simulink model "hps"  (R2021b)
settings: Solver=FixedStepAuto  StartTime=0.0  StopTime=20  FixedStep=0.00909  MaxStep=0.01  RelTol=1e-4  EnableMultiTasking=on
libraries: simulink_extras x5, slpidlib x3, vrlib x3, aerolibutil x2, shared6dof x1, sharedutil x1, sharedtransform x1
settings Model: Creator=rizo  LastModifiedBy=rizo
settings DataIOCC: LimitDataPoints=on  SaveOutput=off  SaveTime=off
settings OptimizationCC: ExpressionDepthLimit=2147483647  LifeSpan=1
settings DebuggingCC: UnderspecifiedInitializationDetection=Classic  MergeDetectMultiDrivingBlocksExec=none  AllowSymbolicDim=off  StateNameClashWarn=warning  SFUnexpectedBacktrackingDiag=warning  SFNoUnconditionalDefaultTransitionDiag=warning  SFExecutionAtInitializationDiag=none  SFMachineParentedDataDiag=warning  ArithmeticOperatorsInVariantConditions=warning
settings SFSimCC: SimUseLocalCustomCode=off  CustomCodeUndefinedFunction=UseInterfaceOnly
settings RTWCC: RTWUseLocalCustomCode=off
settings CodeAppCC: StateflowObjectComments=on
settings GRTTargetCC: TargetLangStandard=C89/C90 (ANSI)  CombineOutputUpdateFcns=off  GRTInterface=on

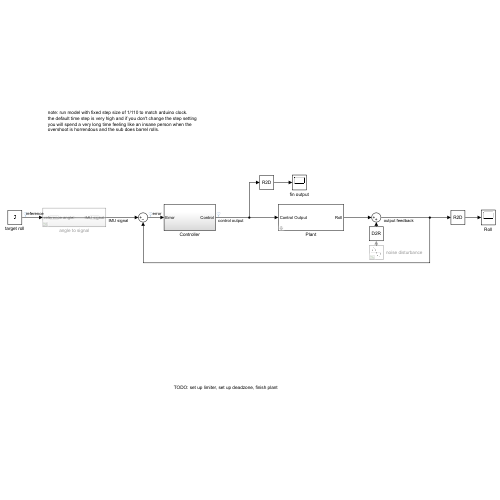
[thumbnail: Simulink's stored preview of the top-level diagram]
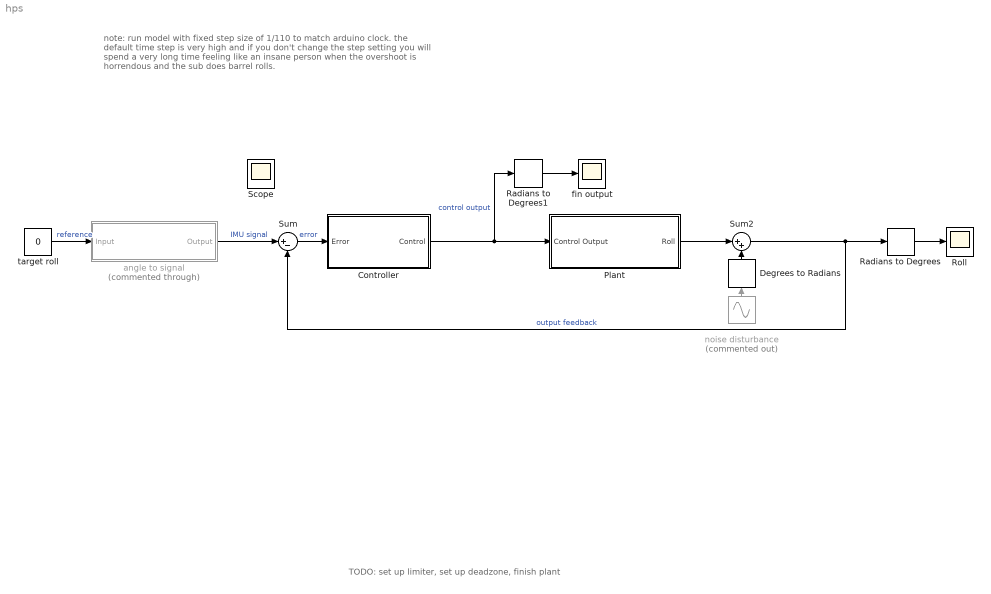
== system hps ==
  note: note: run model with fixed step size of 1/110 to match arduino clock.
      | the default time step is very high and if you don't change the step setting
      | you will spend a very long time feeling like an insane person when the
      | overshoot is horrendous and the sub does barrel rolls.
  note: TODO: set up limiter, set up deadzone, finish plant
  Controller : Subsystem
  Degrees to Radians : simulink_extras/Transformations/Degrees to Radians
  Plant : Subsystem  mask{initial_velocity=1.5, initial_roll=pi/180 * 15, mass=121, Ig=[11.5 -16.5 -21.6; -16.5 165 -3.54; -21.6 -3.54 162], pedaling=10, acc=.25}
      mask prompts: initial_velocity "Initial Velocity"; initial_roll "Initial Roll Angle"; mass "Submarine Mass"; Ig "Inertia matrix"; pedaling "Pedaling Disturbance (N)"; acc "Accerleration (m/s^2)"
  Radians to Degrees : simulink_extras/Transformations/Radians to Degrees
  Radians to Degrees1 : simulink_extras/Transformations/Radians to Degrees
  Roll : Scope
  Sum : Sum  Inputs=|+-
  Sum2 : Sum  Inputs=|++
  angle to signal : Subsystem  Commented=through
  fin output : Scope
  noise disturbance : Sin  Commented=on  Amplitude=0  SampleTime=0
  target roll : Constant  Value=0
  Scope : Scope
  wires:
  target roll/1 -> angle to signal/1(Input)  "reference"
  Sum/1 -> Controller/1(Error)  "error"
  Controller/1(Control) -> Plant/1(Control Output), Radians to Degrees1/1  "control output"
  Sum2/1 -> Sum/2, Radians to Degrees/1  "output feedback"
  angle to signal/1(Output) -> Sum/1  "IMU signal"
  Plant/1(Roll) -> Sum2/1
  Radians to Degrees1/1 -> fin output/1
  Radians to Degrees/1 -> Roll/1
  Degrees to Radians/1 -> Sum2/2
  noise disturbance/1 -> Degrees to Radians/1

== system hps/Controller ==
  Error : Inport
  Controller V0.1 : Subsystem  Commented=on
  Controller V0.2 : Subsystem
  Steering Gear : TransferFcn  Denominator=[1 1]
  Control : Outport
  wires:
  Error/1 -> Controller V0.1/1(Error), Controller V0.2/1(Error)
  Controller V0.2/1(Control) -> Steering Gear/1
  Steering Gear/1 -> Control/1

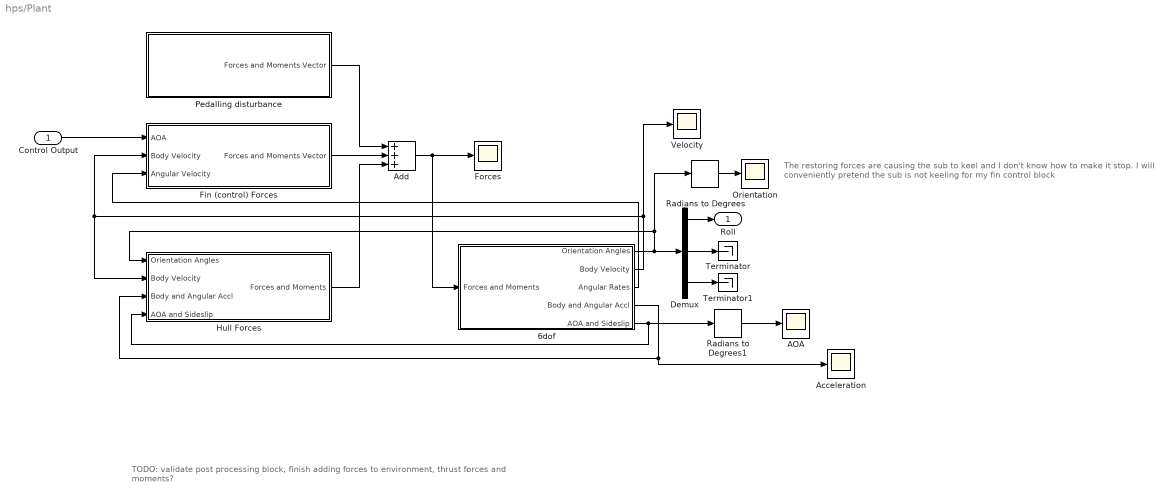
== system hps/Plant ==
  note: The restoring forces are causing the sub to keel and I don't know how to make it stop. I will conveniently pretend the sub is not keeling for my fin control block
  note: TODO: validate post processing block, finish adding forces to environment, thrust forces and moments?
  Control Output : Inport
  6dof : Subsystem
  AOA : Scope
  Acceleration : Scope
  Add : Sum  Inputs=+++
  Demux : Demux  Outputs=3
  Fin (control) Forces : Subsystem  mask{r=.405, finbeam=1.37, semi_major=48.64, semi_minor=12.34, cd=1.28, cl=.108, A=.0942, ro=997}
      mask prompts: r "Fin radius from center"; finbeam "Fin beam"; semi_major "Semi-major axis"; semi_minor "Semi-minor axis"; cd "Coefficient of Drag"; cl "Coefficient of Lift"; A "Planform Area of Wing (m^2)"; ro "Density of Water (kg/m^3)"
  Forces : Scope
  Hull Forces : Subsystem
  Orientation : Scope
  Pedalling disturbance : Subsystem  mask{f=pedaling, a=acc}
      mask prompts: f "Pedal Force (N)"; a "Acceleration (m/s^2)"
  Radians to Degrees : simulink_extras/Transformations/Radians to Degrees
  Radians to Degrees1 : simulink_extras/Transformations/Radians to Degrees
  Terminator : Terminator
  Terminator1 : Terminator
  Velocity : Scope
  Roll : Outport
  wires:
  Control Output/1 -> Fin (control) Forces/1(AOA)
  6dof/1(Orientation Angles) -> Demux/1, Radians to Degrees/1, Hull Forces/1(Orientation Angles)
  Hull Forces/1(Forces and Moments) -> Add/3
  Demux/1 -> Roll/1
  Demux/2 -> Terminator/1
  Demux/3 -> Terminator1/1
  6dof/2(Body Velocity) -> Velocity/1, Hull Forces/2(Body Velocity), Fin (control) Forces/2(Body Velocity)
  Fin (control) Forces/1(Forces and Moments Vector) -> Add/2
  Add/1 -> Forces/1, 6dof/1(Forces and Moments)
  6dof/3(Angular Rates) -> Fin (control) Forces/3(Angular Velocity)
  Pedalling disturbance/1(Forces and Moments Vector) -> Add/1
  6dof/5(AOA and Sideslip) -> Hull Forces/4(AOA and Sideslip), Radians to Degrees1/1
  6dof/4(Body and Angular Accl) -> Acceleration/1, Hull Forces/3(Body and Angular Accl)
  Radians to Degrees/1 -> Orientation/1
  Radians to Degrees1/1 -> AOA/1

== system hps/angle to signal ==
  Input : Inport
  Gain : Gain
  Output : Outport
  wires:
  Gain/1 -> Output/1  "IMU signal"
  Input/1 -> Gain/1  "reference angle"

== system hps/Controller/Controller V0.1 ==
  Error : Inport
  Dead Zone1 : DeadZone  LowerValue=-pi/180 * 2  UpperValue=pi/180 * 2  SaturateOnIntegerOverflow=on
  Dead Zone2 : DeadZone  LowerValue=-pi/180 * 2  UpperValue=pi/180 * 2  SaturateOnIntegerOverflow=on
  PI Controller : slpidlib/PID Controller  Controller=PID  Form=Parallel  TimeDomain=Continuous-time  UseExternalTs=off  SampleTime=-1  IntegratorMethod=Forward Euler  FilterMethod=Forward Euler  ControllerParametersSource=internal  P=4  I=1  D=0  UseFilter=on  N=100  TunerSelectOption=Transfer Function Based (PID Tuner App)  InitialConditionSource=internal  InitialConditionForIntegrator=0  InitialConditionForFilter=0  DifferentiatorICPrevScaledInput=0  ExternalReset=none  TrackingMode=off  Kt=1  LimitOutput=off  SatLimitsSource=internal  UpperSaturationLimit=inf  LowerSaturationLimit=-inf  LinearizeAsGain=on  AntiWindupMode=none  Kb=1  POutMin=[]  POutMax=[]  IOutMin=[]  IOutMax=[]  DOutMin=[]  DOutMax=[]  NOutMin=[]  NOutMax=[]  SumOutMin=[]  SumOutMax=[]  SaturationOutMin=[]  SaturationOutMax=[]  PParamMin=[]  PParamMax=[]  IParamMin=[]  IParamMax=[]  DParamMin=[]  DParamMax=[]  NParamMin=[]  NParamMax=[]  KbParamMin=[]  KbParamMax=[]  KtParamMin=[]  KtParamMax=[]  KbOutMin=[]  KbOutMax=[]  KtOutMin=[]  KtOutMax=[]  IntegratorOutMin=[]  IntegratorOutMax=[]  FilterOutMin=[]  FilterOutMax=[]  SumI1OutMin=[]  SumI1OutMax=[]  SumI2OutMin=[]  SumI2OutMax=[]  SumI3OutMin=[]  SumI3OutMax=[]  SumI4OutMin=[]  SumI4OutMax=[]  SumDOutMin=[]  SumDOutMax=[]  DifferentiatorOutMin=[]  DifferentiatorOutMax=[]  FilterDiffOutCoefMin=[]  FilterDiffOutCoefMax=[]  ReciprocalOutMin=[]  ReciprocalOutMax=[]  SumDenOutMin=[]  SumDenOutMax=[]  SumNumOutMin=[]  SumNumOutMax=[]  DivideOutMin=[]  DivideOutMax=[]  UdiffTsProdOutMin=[]  UdiffTsProdOutMax=[]  NTsProdOutMin=[]  NTsProdOutMax=[]  UintegralTsProdOutMin=[]  UintegralTsProdOutMax=[]  UngainTsProdOutMin=[]  UngainTsProdOutMax=[]  IntegratorContinuousStateAttributes=''  IntegratorStateMustResolveToSignalObject=off  IntegratorRTWStateStorageClass=Auto  FilterContinuousStateAttributes=''  FilterStateMustResolveToSignalObject=off  FilterRTWStateStorageClass=Auto  ParallelPVariant=InternalParameters  IdealPVariant=Disabled  IVariant=InternalParameters  DVariant=InternalParameters  IntegratorVariant=Continuous  SatVariant=Disabled  AWVariant=Passthrough  PCopyVariant=Disabled  TRVariant=Disabled  FdbkBlocksVariant=Forward  IdealPFdbkVariant=Disabled  SatFdbkVariant=Disabled  DerivativeFilterVariant=ContFilter  NVariant=InternalParameters  NCopyVariant=Disabled  FilterICVariant=InternalICsFilter  IntegratorICVariant=InternalICs  ExternalResetVariant=Disabled  TRSumVariant=Passthrough  SumFdbkVariant=Disabled  SumVariant=Sum_PID  TsampFilterVariant=InternalTs  TsampNgainVariant=Passthrough  TsampIntegralVariant=Passthrough  ExternalSaturationOutDataTypeStr=Inherit: Same as second input
  PID Controller : slpidlib/PID Controller  Controller=PID  Form=Parallel  TimeDomain=Continuous-time  UseExternalTs=off  SampleTime=-1  IntegratorMethod=Forward Euler  FilterMethod=Forward Euler  ControllerParametersSource=internal  P=4  I=2  D=1  UseFilter=on  N=100  TunerSelectOption=Transfer Function Based (PID Tuner App)  InitialConditionSource=internal  InitialConditionForIntegrator=0  InitialConditionForFilter=0  DifferentiatorICPrevScaledInput=0  ExternalReset=none  TrackingMode=off  Kt=1  LimitOutput=off  SatLimitsSource=internal  UpperSaturationLimit=inf  LowerSaturationLimit=-inf  LinearizeAsGain=on  AntiWindupMode=none  Kb=1  POutMin=[]  POutMax=[]  IOutMin=[]  IOutMax=[]  DOutMin=[]  DOutMax=[]  NOutMin=[]  NOutMax=[]  SumOutMin=[]  SumOutMax=[]  SaturationOutMin=[]  SaturationOutMax=[]  PParamMin=[]  PParamMax=[]  IParamMin=[]  IParamMax=[]  DParamMin=[]  DParamMax=[]  NParamMin=[]  NParamMax=[]  KbParamMin=[]  KbParamMax=[]  KtParamMin=[]  KtParamMax=[]  KbOutMin=[]  KbOutMax=[]  KtOutMin=[]  KtOutMax=[]  IntegratorOutMin=[]  IntegratorOutMax=[]  FilterOutMin=[]  FilterOutMax=[]  SumI1OutMin=[]  SumI1OutMax=[]  SumI2OutMin=[]  SumI2OutMax=[]  SumI3OutMin=[]  SumI3OutMax=[]  SumI4OutMin=[]  SumI4OutMax=[]  SumDOutMin=[]  SumDOutMax=[]  DifferentiatorOutMin=[]  DifferentiatorOutMax=[]  FilterDiffOutCoefMin=[]  FilterDiffOutCoefMax=[]  ReciprocalOutMin=[]  ReciprocalOutMax=[]  SumDenOutMin=[]  SumDenOutMax=[]  SumNumOutMin=[]  SumNumOutMax=[]  DivideOutMin=[]  DivideOutMax=[]  UdiffTsProdOutMin=[]  UdiffTsProdOutMax=[]  NTsProdOutMin=[]  NTsProdOutMax=[]  UintegralTsProdOutMin=[]  UintegralTsProdOutMax=[]  UngainTsProdOutMin=[]  UngainTsProdOutMax=[]  IntegratorContinuousStateAttributes=''  IntegratorStateMustResolveToSignalObject=off  IntegratorRTWStateStorageClass=Auto  FilterContinuousStateAttributes=''  FilterStateMustResolveToSignalObject=off  FilterRTWStateStorageClass=Auto  ParallelPVariant=InternalParameters  IdealPVariant=Disabled  IVariant=InternalParameters  DVariant=InternalParameters  IntegratorVariant=Continuous  SatVariant=Disabled  AWVariant=Passthrough  PCopyVariant=Disabled  TRVariant=Disabled  FdbkBlocksVariant=Forward  IdealPFdbkVariant=Disabled  SatFdbkVariant=Disabled  DerivativeFilterVariant=ContFilter  NVariant=InternalParameters  NCopyVariant=Disabled  FilterICVariant=InternalICsFilter  IntegratorICVariant=InternalICs  ExternalResetVariant=Disabled  TRSumVariant=Passthrough  SumFdbkVariant=Disabled  SumVariant=Sum_PID  TsampFilterVariant=InternalTs  TsampNgainVariant=Passthrough  TsampIntegralVariant=Passthrough  ExternalSaturationOutDataTypeStr=Inherit: Same as second input
  Saturation : Saturate  UpperLimit=pi/4  LowerLimit=-pi/4
  Saturation1 : Saturate  UpperLimit=pi/4  LowerLimit=-pi/4
  Sum : Sum  Inputs=|+-
  Transfer Fcn : TransferFcn  Denominator=[1 1]
  Control : Outport
  wires:
  Error/1 -> PID Controller/1
  Sum/1 -> PI Controller/1
  PI Controller/1 -> Saturation1/1
  Saturation1/1 -> Dead Zone2/1
  PID Controller/1 -> Saturation/1
  Saturation/1 -> Dead Zone1/1
  Dead Zone1/1 -> Sum/1
  Dead Zone2/1 -> Transfer Fcn/1
  Transfer Fcn/1 -> Sum/2, Control/1

== system hps/Controller/Controller V0.2 ==
  Error : Inport
  Dead Zone : DeadZone  LowerValue=-pi/180 * 2  UpperValue=pi/180 * 2  SaturateOnIntegerOverflow=on
  IC : InitialCondition  Value=0
  PID : slpidlib/PID Controller  Controller=PID  Form=Parallel  TimeDomain=Discrete-time  UseExternalTs=off  SampleTime=-1  IntegratorMethod=Forward Euler  FilterMethod=Forward Euler  ControllerParametersSource=internal  P=5  I=0.1  D=10  UseFilter=off  N=3  TunerSelectOption=Transfer Function Based (PID Tuner App)  InitialConditionSource=internal  InitialConditionForIntegrator=0  InitialConditionForFilter=0  DifferentiatorICPrevScaledInput=0  ExternalReset=none  TrackingMode=off  Kt=1  LimitOutput=off  SatLimitsSource=internal  UpperSaturationLimit=pi/18  LowerSaturationLimit=-pi/18  LinearizeAsGain=on  AntiWindupMode=none  Kb=1  POutMin=[]  POutMax=[]  IOutMin=[]  IOutMax=[]  DOutMin=[]  DOutMax=[]  NOutMin=[]  NOutMax=[]  SumOutMin=[]  SumOutMax=[]  SaturationOutMin=[]  SaturationOutMax=[]  PParamMin=[]  PParamMax=[]  IParamMin=[]  IParamMax=[]  DParamMin=[]  DParamMax=[]  NParamMin=[]  NParamMax=[]  KbParamMin=[]  KbParamMax=[]  KtParamMin=[]  KtParamMax=[]  KbOutMin=[]  KbOutMax=[]  KtOutMin=[]  KtOutMax=[]  IntegratorOutMin=[]  IntegratorOutMax=[]  FilterOutMin=[]  FilterOutMax=[]  SumI1OutMin=[]  SumI1OutMax=[]  SumI2OutMin=[]  SumI2OutMax=[]  SumI3OutMin=[]  SumI3OutMax=[]  SumI4OutMin=[]  SumI4OutMax=[]  SumDOutMin=[]  SumDOutMax=[]  DifferentiatorOutMin=[]  DifferentiatorOutMax=[]  FilterDiffOutCoefMin=[]  FilterDiffOutCoefMax=[]  ReciprocalOutMin=[]  ReciprocalOutMax=[]  SumDenOutMin=[]  SumDenOutMax=[]  SumNumOutMin=[]  SumNumOutMax=[]  DivideOutMin=[]  DivideOutMax=[]  UdiffTsProdOutMin=[]  UdiffTsProdOutMax=[]  NTsProdOutMin=[]  NTsProdOutMax=[]  UintegralTsProdOutMin=[]  UintegralTsProdOutMax=[]  UngainTsProdOutMin=[]  UngainTsProdOutMax=[]  IntegratorContinuousStateAttributes=''  IntegratorStateMustResolveToSignalObject=off  IntegratorRTWStateStorageClass=Auto  FilterContinuousStateAttributes=''  FilterStateMustResolveToSignalObject=off  FilterRTWStateStorageClass=Auto  ParallelPVariant=InternalParameters  IdealPVariant=Disabled  IVariant=InternalParameters  DVariant=InternalParameters  IntegratorVariant=Discrete  SatVariant=Disabled  AWVariant=Passthrough  PCopyVariant=Disabled  TRVariant=Disabled  FdbkBlocksVariant=Forward  IdealPFdbkVariant=Disabled  SatFdbkVariant=Disabled  DerivativeFilterVariant=Differentiator  NVariant=Passthrough  NCopyVariant=Disabled_SignalSpec  FilterICVariant=InternalICsDifferentiator  IntegratorICVariant=InternalICs  ExternalResetVariant=Disabled  TRSumVariant=Passthrough  SumFdbkVariant=Disabled  SumVariant=Sum_PID  TsampFilterVariant=InternalTs  TsampNgainVariant=Passthrough  TsampIntegralVariant=Passthrough  ExternalSaturationOutDataTypeStr=Inherit: Same as second input
  Saturation : Saturate  UpperLimit=pi/18  LowerLimit=-pi/18
  Steering gear : TransferFcn  Commented=through  Denominator=[1 1]
  Control : Outport
  wires:
  Saturation/1 -> Steering gear/1
  PID/1 -> IC/1
  IC/1 -> Saturation/1
  Error/1 -> Dead Zone/1
  Dead Zone/1 -> PID/1
  Steering gear/1 -> Control/1

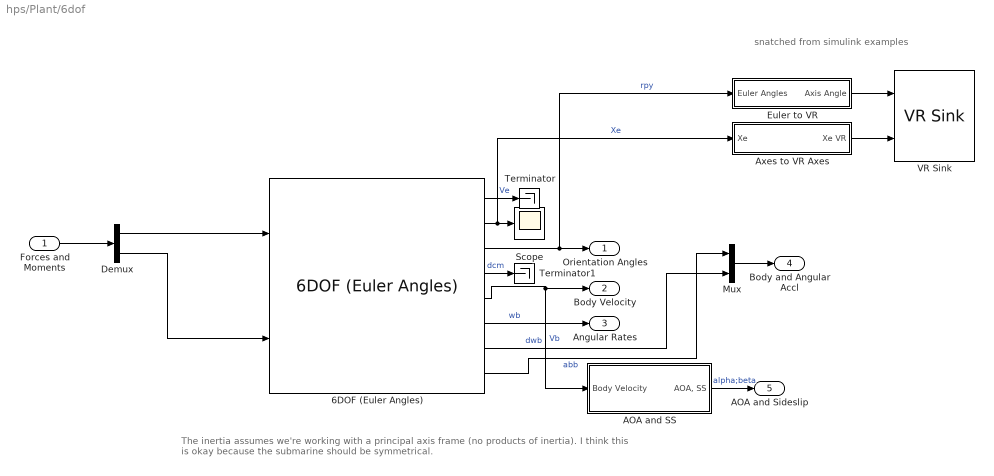
== system hps/Plant/6dof ==
  note: snatched from simulink examples
  note: The inertia assumes we're working with a principal axis frame (no products of inertia). I think this is okay because the submarine should be symmetrical.
  Forces and Moments : Inport
  6DOF (Euler Angles) : shared6dof/6DOF (Euler Angles)  units=Metric (MKS)  mtype=Fixed  rep=Euler Angles  xme_0=[0 0 0]  Vm_0=[initial_velocity 0 0]  eul_0=[initial_roll 0 0]  pm_0=[0 0 0]  mass_0=mass  mass_e=0.5  mass_f=2.0  inertia=mass * eye(3)  inertia_e=eye(3)  inertia_f=2*eye(3)  k_quat=1.0  vre_flag=on  abi_flag=off  aMode=0  xme_statename=''  Vm_statename=''  eul_statename=''  quat_statename=''  pm_statename=''  mass_statename=''
      settings: SourceProductBaseCode=AE,PW,DR,MT,UV,VE
  AOA and SS : Subsystem
  Axes to VR Axes : Subsystem
  Demux : Demux  Outputs=2
  Euler to VR : Subsystem
  Mux : Mux  Inputs=2
  Scope : Scope
  Terminator : Terminator
  Terminator1 : Terminator
  VR Sink : vrlib/VR Sink  InstantiateOnLoad=on  SampleTime=0.00909  ViewEnable=on  RemoteChange=off  RemoteView=off  FieldsWritten=HL20.rotation.4.1.1.double#HL20.translation.3.1.1.double  WorldFileName=aeroblk_HL20.wrl  WorldDescription=aeroblk_HL20  AutoView=on  VideoDimensions=[]  AllowVariableSize=off
  Orientation Angles : Outport
  Body Velocity : Outport  Port=2
  Angular Rates : Outport  Port=3
  Body and Angular Accl : Outport  Port=4
  AOA and Sideslip : Outport  Port=5
  wires:
  Forces and Moments/1 -> Demux/1
  Demux/1 -> 6DOF (Euler Angles)/1
  Demux/2 -> 6DOF (Euler Angles)/2
  6DOF (Euler Angles)/6 -> Angular Rates/1  "wb"
  6DOF (Euler Angles)/7 -> Mux/2  "dwb"
  6DOF (Euler Angles)/8 -> Mux/1  "abb"
  6DOF (Euler Angles)/2 -> Axes to VR Axes/1(Xe), Scope/1  "Xe"
  6DOF (Euler Angles)/3 -> Euler to VR/1(Euler Angles), Orientation Angles/1  "rpy"
  6DOF (Euler Angles)/5 -> AOA and SS/1(Body Velocity), Body Velocity/1  "Vb"
  AOA and SS/1("AOA, SS") -> AOA and Sideslip/1  "alpha;beta"
  Mux/1 -> Body and Angular Accl/1
  Axes to VR Axes/1(Xe VR) -> VR Sink/2
  Euler to VR/1(Axis Angle) -> VR Sink/1
  6DOF (Euler Angles)/1 -> Terminator/1  "Ve"
  6DOF (Euler Angles)/4 -> Terminator1/1  "dcm"

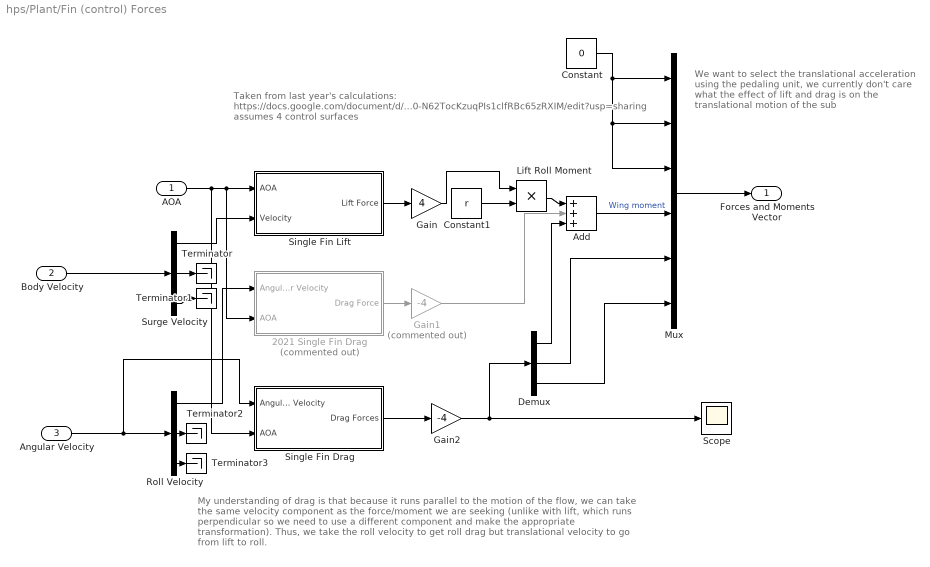
== system hps/Plant/Fin (control) Forces ==
  note: We want to select the translational acceleration using the pedaling unit, we currently don't care what the effect of lift and drag is on the translational motion of the sub
  note: My understanding of drag is that because it runs parallel to the motion of the flow, we can take the same velocity component as the force/moment we are seeking (unlike with lift, which runs perpendicular so we need to use a different component and make the appropriate transformation). Thus, we take the roll velocity to get roll drag but translational velocity to go from lift to roll.
  note: Taken from last year's calculations:
      | https://docs.google.com/document/d/1lyuNGJgZCwyaSb0-N62TocKzuqPIs1clfRBc65zRXIM/edit?usp=sharing
      |
      | assumes 4 control surfaces
  AOA : Inport
  Body Velocity : Inport  Port=2
  Angular Velocity : Inport  Port=3
  2021 Single Fin Drag : Subsystem  Commented=on
  Add : Sum  Inputs=+++
  Constant : Constant  Value=0
  Constant1 : Constant  Value=r
  Demux : Demux  Outputs=3
  Gain : Gain  Gain=4
  Gain1 : Gain  Commented=on  Gain=-4
  Gain2 : Gain  Gain=-4
  Lift Roll Moment : Product
  Mux : Mux  Inputs=6
  Roll Velocity : Demux  Outputs=3
  Scope : Scope
  Single Fin Drag : Subsystem
  Single Fin Lift : Subsystem
  Surge Velocity : Demux  Outputs=3
  Terminator{,1..3} (4 alike) : Terminator
  Forces and Moments Vector : Outport
  wires:
  Single Fin Lift/1(Lift Force) -> Gain/1
  Constant/1 -> Mux/3, Mux/2, Mux/1
  Mux/1 -> Forces and Moments Vector/1
  AOA/1 -> Single Fin Drag/2(AOA), 2021 Single Fin Drag/2(AOA), Single Fin Lift/1(AOA)
  Gain/1 -> Lift Roll Moment/1
  Constant1/1 -> Lift Roll Moment/2
  Body Velocity/1 -> Surge Velocity/1
  Surge Velocity/2 -> Terminator/1
  Surge Velocity/3 -> Terminator1/1
  Surge Velocity/1 -> Single Fin Lift/2(Velocity)
  Angular Velocity/1 -> Single Fin Drag/1(Angular Velocity), Roll Velocity/1
  Roll Velocity/2 -> Terminator2/1
  Roll Velocity/3 -> Terminator3/1
  Roll Velocity/1 -> 2021 Single Fin Drag/1(Angular Velocity)
  2021 Single Fin Drag/1(Drag Force) -> Gain1/1
  Gain1/1 -> Add/2
  Lift Roll Moment/1 -> Add/1
  Add/1 -> Mux/4  "Wing moment"
  Single Fin Drag/1(Drag Forces) -> Gain2/1
  Gain2/1 -> Demux/1, Scope/1
  Demux/3 -> Mux/6
  Demux/2 -> Mux/5
  Demux/1 -> Add/3

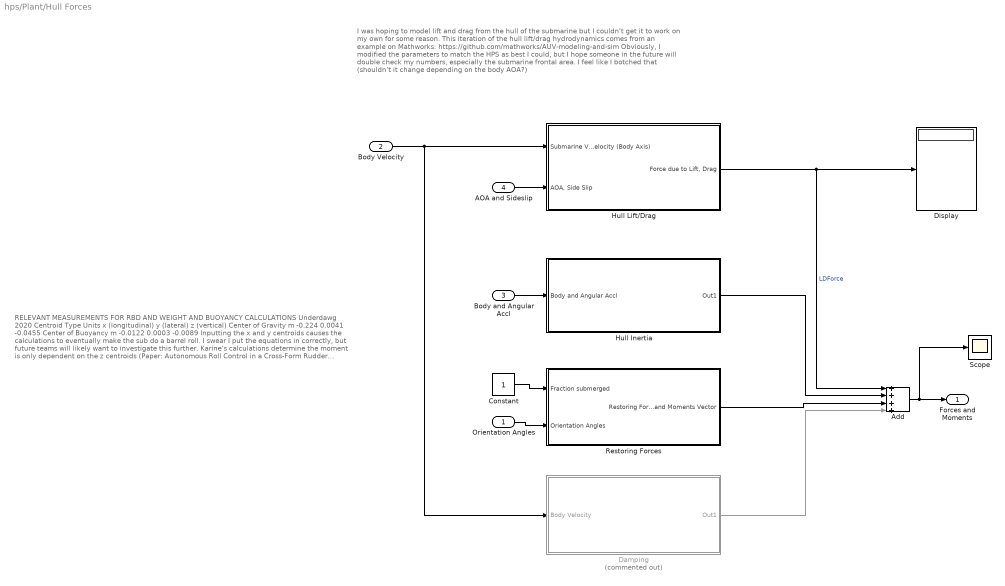
== system hps/Plant/Hull Forces ==
  note: I was hoping to model lift and drag from the hull of the submarine but I couldn't get it to work on my own for some reason. This iteration of the hull lift/drag hydrodynamics comes from an example on Mathworks: https://github.com/mathworks/AUV-modeling-and-sim
      |
      | Obviously, I modified the parameters to match the HPS as best I could, but I hope someone in the future will double check my numbers, especially the submarine frontal area. I feel like I botched that (shouldn't it change depending on the body AOA?)
  note: RELEVANT MEASUREMENTS FOR RBD AND WEIGHT AND BUOYANCY CALCULATIONS
      |
      | Underdawg 2020
      | Centroid Type Units x (longitudinal) y (lateral) z (vertical)
      | Center of Gravity m -0.224 0.0041 -0.0455
      | Center of Buoyancy m -0.0122 0.0003 -0.0089
      |
      | Inputting the x and y centroids causes the calculations to eventually make the sub do a barrel roll.
      | I swear I put the equations in correctly, but future teams will likely want to investigate this further. Karine's calculations determine the moment is only dependent on the z centroids (Paper: Autonomous Roll Control in a Cross-Form Rudder Submarine Using PID Controllers, section 3.7, eq 3.37), so the x and y centroids are set to 0 for equations that need them.
  Orientation Angles : Inport
  Body Velocity : Inport  Port=2
  Body and Angular Accl : Inport  Port=3
  AOA and Sideslip : Inport  Port=4
  Add : Sum  Inputs=++++
  Constant : Constant
  Damping : Subsystem  Commented=on
  Display : Display
  Hull Inertia : Subsystem
  Hull Lift/Drag : Subsystem  VariantControl=c==1
  Restoring Forces : Subsystem  mask{ro=997, V=0.122, M=mass, CGx=0, CGy=0, CGz=0.0455, CBx=0, CBy=0, CBz=0.0089}
      mask prompts: ro "Density of Water"; V "Volume of Submarine"; M "Mass of Submarine"
      mask DialogControl DescTextVar Prompt: Enter the Submarine related Parameters
      mask DialogControl Container3 Prompt: Centroids
  Scope : Scope
  Forces and Moments : Outport
  wires:
  Orientation Angles/1 -> Restoring Forces/2(Orientation Angles)
  Add/1 -> Forces and Moments/1, Scope/1
  Restoring Forces/1(Restoring Forces and Moments Vector) -> Add/3
  AOA and Sideslip/1 -> Hull Lift/Drag/2("AOA, Side Slip")
  Hull Inertia/1(Out1) -> Add/2
  Body Velocity/1 -> Hull Lift/Drag/1("Submarine Velocity (Body Axis) "), Damping/1(Body Velocity)
  Body and Angular Accl/1 -> Hull Inertia/1(Body and Angular Accl)
  Hull Lift/Drag/1("Force due to Lift, Drag") -> Display/1, Add/1  "LDForce"
  Damping/1(Out1) -> Add/4
  Constant/1 -> Restoring Forces/1("Fraction submerged ")

== system hps/Plant/Pedalling disturbance ==
  note: https://thebodymechanic.com.au/cycling-cadence-what-is-it-and-why-you-should-keep-a-close-eye-on-yours/
      |
      | "advanced and elite cyclists pedal anywhere from 90 to 110 RPM."
      |
      | Current cycle rate is 90 RPM, assuming an advanced cyclist's pedal rate is similar to the HPS pilot's pedal rate
  Acceleration force : Constant  Value=mass*a
  Constant : Constant  Value=0
  Mux : Mux  Inputs=6
  Pedalling : Sin  Amplitude=f  Frequency=2*pi * 90/60  SampleTime=0
  Forces and Moments Vector : Outport
  wires:
  Mux/1 -> Forces and Moments Vector/1
  Constant/1 -> Mux/5, Mux/3, Mux/2, Mux/6
  Pedalling/1 -> Mux/4
  Acceleration force/1 -> Mux/1

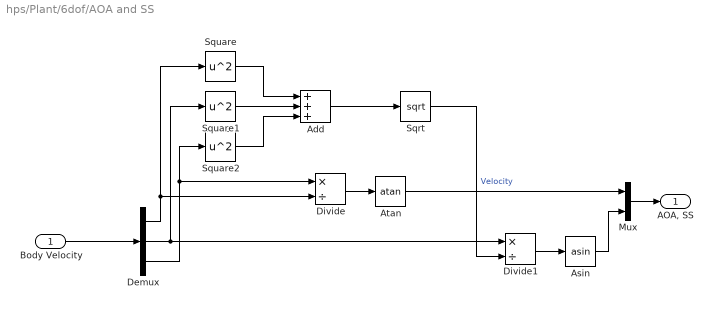
== system hps/Plant/6dof/AOA and SS ==
  Body Velocity : Inport
  Add : Sum  Inputs=+++
  Asin : Trigonometry  Operator=asin
  Atan : Trigonometry  Operator=atan
  Demux : Demux  Outputs=3
  Divide : Product  Inputs=*/
  Divide1 : Product  Inputs=*/
  Mux : Mux  Inputs=2
  Sqrt : Sqrt  SaturateOnIntegerOverflow=on
  Square : Math  Operator=square  SaturateOnIntegerOverflow=on
  Square1 : Math  Operator=square  SaturateOnIntegerOverflow=on
  Square2 : Math  Operator=square  SaturateOnIntegerOverflow=on
  "AOA, SS" : Outport
  wires:
  Body Velocity/1 -> Demux/1
  Demux/1 -> Divide/2, Square/1
  Demux/2 -> Square1/1, Divide1/1
  Demux/3 -> Divide/1, Square2/1
  Add/1 -> Sqrt/1
  Square/1 -> Add/1
  Square1/1 -> Add/2
  Square2/1 -> Add/3
  Sqrt/1 -> Divide1/2  "Velocity"
  Divide/1 -> Atan/1
  Divide1/1 -> Asin/1
  Atan/1 -> Mux/1
  Asin/1 -> Mux/2
  Mux/1 -> "AOA, SS"/1

== system hps/Plant/6dof/Axes to VR Axes ==
  Xe : Inport
  Concatenate : Concatenate  NumInputs=3
  Demux : Demux  Outputs=3
      settings: DisplayOption=none
  rad-->deg : Gain  Gain=-1  SaturateOnIntegerOverflow=on  OutDataTypeStr=Inherit: Same as input  ParamDataTypeStr=Inherit: Same as input
  rad-->deg1 : Gain  Gain=-1  SaturateOnIntegerOverflow=on  OutDataTypeStr=Inherit: Same as input  ParamDataTypeStr=Inherit: Same as input
  Xe VR : Outport  VectorParamsAs1DForOutWhenUnconnected=off
  wires:
  Xe/1 -> Demux/1
  Demux/1 -> Concatenate/1
  Demux/2 -> rad-->deg/1
  Demux/3 -> rad-->deg1/1
  Concatenate/1 -> Xe VR/1
  rad-->deg1/1 -> Concatenate/2
  rad-->deg/1 -> Concatenate/3

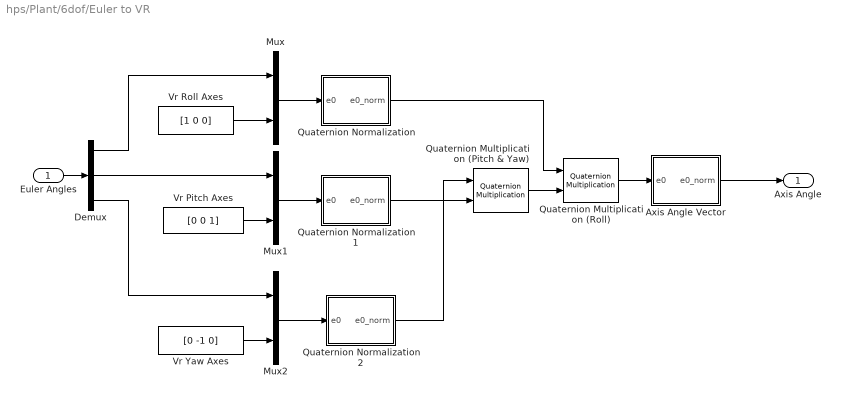
== system hps/Plant/6dof/Euler to VR ==
  Euler Angles : Inport
  Axis Angle Vector : Subsystem
  Demux : Demux  Outputs=3
      settings: DisplayOption=none
  Mux : Mux  Inputs=2
  Mux1 : Mux  Inputs=2
  Mux2 : Mux  Inputs=2
  Quaternion Multiplication (Pitch & Yaw) : aerolibutil/Quaternion Multiplication
  Quaternion Multiplication (Roll) : aerolibutil/Quaternion Multiplication
  Quaternion Normalization : Subsystem
  Quaternion Normalization1 : Subsystem
  Quaternion Normalization2 : Subsystem
  Vr Pitch Axes : Constant  Value=[0 0 1]
  Vr Roll Axes : Constant  Value=[1 0 0]
  Vr Yaw Axes : Constant  Value=[0 -1 0]
  Axis Angle : Outport  VectorParamsAs1DForOutWhenUnconnected=off
  wires:
  Quaternion Multiplication (Roll)/1 -> Axis Angle Vector/1(e0)
  Quaternion Multiplication (Pitch & Yaw)/1 -> Quaternion Multiplication (Roll)/2
  Axis Angle Vector/1(e0_norm) -> Axis Angle/1
  Quaternion Normalization/1(e0_norm) -> Quaternion Multiplication (Roll)/1
  Quaternion Normalization2/1(e0_norm) -> Quaternion Multiplication (Pitch & Yaw)/1
  Quaternion Normalization1/1(e0_norm) -> Quaternion Multiplication (Pitch & Yaw)/2
  Mux2/1 -> Quaternion Normalization2/1(e0)
  Mux1/1 -> Quaternion Normalization1/1(e0)
  Mux/1 -> Quaternion Normalization/1(e0)
  Demux/3 -> Mux2/1
  Vr Yaw Axes/1 -> Mux2/2
  Demux/2 -> Mux1/1
  Vr Pitch Axes/1 -> Mux1/2
  Demux/1 -> Mux/1
  Vr Roll Axes/1 -> Mux/2
  Euler Angles/1 -> Demux/1

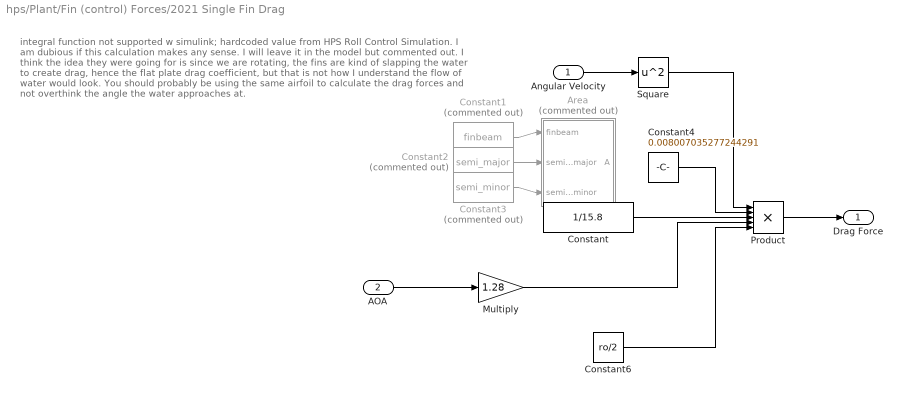
== system hps/Plant/Fin (control) Forces/2021 Single Fin Drag ==
  note: integral function not supported w simulink; hardcoded value from HPS Roll Control Simulation. I am dubious if this calculation makes any sense. I will leave it in the model but commented out. I think the idea they were going for is since we are rotating, the fins are kind of slapping the water to create drag, hence the flat plate drag coefficient, but that is not how I understand the flow of water would look. You should probably be using the same airfoil to calculate the drag forces and not overthink the angle the water approaches at.
  Angular Velocity : Inport
  AOA : Inport  Port=2
  Area : MATLAB Function  Commented=on  TreatAsAtomicUnit=on
  Constant : Constant  Value=1/15.8
  Constant1 : Constant  Commented=on  Value=finbeam
  Constant2 : Constant  Commented=on  Value=semi_major
  Constant3 : Constant  Commented=on  Value=semi_minor
  Constant4 : Constant  Value=0.008007035277244291
  Constant6 : Constant  Value=ro/2
  Multiply : Gain  Gain=1.28
  Product : Product  Inputs=5
  Square : Math  Operator=square  SaturateOnIntegerOverflow=on
  Drag Force : Outport
  wires:
  Constant1/1 -> Area/1(finbeam)
  Constant3/1 -> Area/3(semi_minor)
  Constant2/1 -> Area/2(semi_major)
  Angular Velocity/1 -> Square/1
  Constant/1 -> Product/3
  Square/1 -> Product/1
  Multiply/1 -> Product/4
  Constant6/1 -> Product/5
  Product/1 -> Drag Force/1
  Constant4/1 -> Product/2
  AOA/1 -> Multiply/1

== system hps/Plant/Fin (control) Forces/Single Fin Drag ==
  Angular Velocity : Inport
  AOA : Inport  Port=2
  Constant1 : Constant  Value=ro
  Constant2 : Constant  Value=A
  Gain : Gain  Gain=1/2
  MATLAB Function1 : MATLAB Function  TreatAsAtomicUnit=on
  Product : Product  Inputs=4
  Saturation1 : Saturate  UpperLimit=56.214  LowerLimit=-56.214
  Square1 : Math  Operator=square  SaturateOnIntegerOverflow=on
  Drag Forces : Outport
  wires:
  AOA/1 -> MATLAB Function1/1(u)
  MATLAB Function1/1(C_D) -> Saturation1/1
  Constant2/1 -> Product/2
  Gain/1 -> Drag Forces/1
  Constant1/1 -> Product/3
  Product/1 -> Gain/1
  Angular Velocity/1 -> Square1/1
  Square1/1 -> Product/1
  Saturation1/1 -> Product/4

== system hps/Plant/Fin (control) Forces/Single Fin Lift ==
  AOA : Inport
  Velocity : Inport  Port=2
  Constant1 : Constant  Value=ro
  Constant2 : Constant  Value=A
  Gain : Gain  Gain=1/2
  MATLAB Function : MATLAB Function  TreatAsAtomicUnit=on
  Product : Product  Inputs=4
  Saturation : Saturate  UpperLimit=56.214  LowerLimit=-56.214
  Square : Math  Operator=square  SaturateOnIntegerOverflow=on
  Lift Force : Outport
  wires:
  Constant1/1 -> Product/3
  Velocity/1 -> Square/1
  Square/1 -> Product/4
  Product/1 -> Gain/1
  Constant2/1 -> Product/2
  AOA/1 -> MATLAB Function/1(u)
  MATLAB Function/1(y) -> Saturation/1
  Saturation/1 -> Product/1
  Gain/1 -> Lift Force/1

== system hps/Plant/Hull Forces/Damping ==
  Body Velocity : Inport
  Out1 : Outport
  wires:
  Body Velocity/1 -> Out1/1

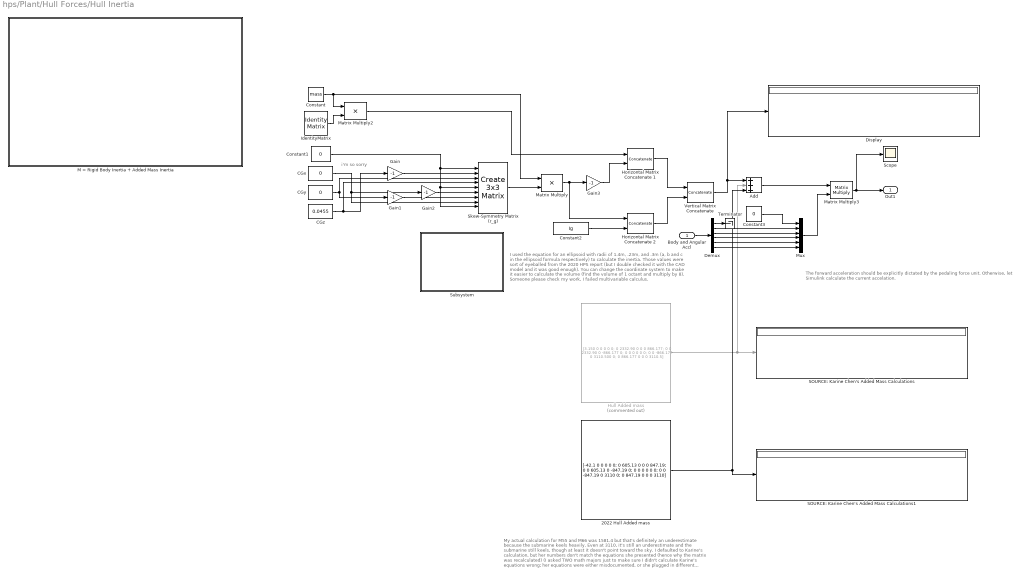
== system hps/Plant/Hull Forces/Hull Inertia ==
  note: My actual calculation for M55 and M66 was 1581.4 but that's definitely an underestimate because the submarine keels heavily. Even at 3110, it's still an underestimate and the submarine still keels, though at least it doesn't point toward the sky. I defaulted to Karine's calculation, but her numbers don't match the equations she presented (hence why the matrix was recalculated) (I asked TWO math majors just to make sure I didn't calculate Karine's equations wrong; her equations were either misdocumented, or she plugged in different numbers than what her tables had because NOTHING came up the same)
  note: The forward acceleration should be explicitly dictated by the pedaling force unit. Otherwise, let Simulink calculate the current accelation.
  note: I used the equation for an ellipsoid with radii of 1.4m, .23m, and .3m (a, b and c in the ellipsoid formula respectively) to calculate the inertia. Those values were sort of eyeballed from the 2020 HPS report (but I double checked it with the CAD model and it was good enough). You can change the coordinate system to make it easier to calculate the volume (find the volume of 1 octant and multiply by 8). Someone please check my work, I failed multivariable calculus.
  note: i'm so sorry
  Body and Angular Accl : Inport
  2022 Hull Added mass : Constant  Value=[-42.1 0 0 0 0 0; 0 605.13 0 0 0 847.19; 0 0 605.13 0 -847.19 0; 0 0 0 0 0 0; 0 0 -847.19 0 3110 0; 0 847.19 0 0 0 3110]
  Add : Sum  Inputs=+++
  CGx : Constant  Value=0
  CGy : Constant  Value=0
  CGz : Constant  Value=0.0455
  Constant : Constant  Value=mass
  Constant1 : Constant  Value=0
  Constant2 : Constant  Value=Ig
  Constant3 : Constant  Value=0
  Demux : Demux  Outputs=6
  Display : Display
  Gain{,1..3} (4 alike) : Gain  Gain=-1
  Horizontal Matrix Concatenate 1 : Concatenate  Mode=Multidimensional array  ConcatenateDimension=2
  Horizontal Matrix Concatenate 2 : Concatenate  Mode=Multidimensional array  ConcatenateDimension=2
  Hull Added mass : Constant  Commented=on  Value=[3.150 0 0 0 0 0; 0 2332.90 0 0 0 866.177; 0 0 2332.90 0 -866.177 0; 0 0 0 0 0 0; 0 0 -866.177 0 3110.500 0; 0 866.177 0 0 0 3110.5]
  IdentityMatrix : IdentityMatrix  OutputDimensions=3  SampleTime=0.00909
  M = Rigid Body Inertia + Added Mass Inertia : Subsystem
      mask Display: image('$imagefile'); % Use "Edit Image" on toolstrip to change.
  Matrix Multiply : Product
  Matrix Multiply2 : Product
  Matrix Multiply3 : Product  Multiplication=Matrix(*)
  Mux : Mux  Inputs=6
  SOURCE: Karine Chen's Added Mass Calculations : Display
  SOURCE: Karine Chen's Added Mass Calculations1 : Display
  Scope : Scope
  Skew-Symmetry Matrix (r_g) : sharedutil/Create 3x3 Matrix  aMode=aMode
      settings: SourceProductBaseCode=AE,PW,DR,MT,UV,VE
  Subsystem : Subsystem
      mask Display: image('$imagefile'); % Use "Edit Image" on toolstrip to change.
  Terminator : Terminator
  Vertical Matrix Concatenate : Concatenate  Mode=Multidimensional array
  Out1 : Outport
  wires:
  Constant/1 -> Matrix Multiply/1, Matrix Multiply2/1
  IdentityMatrix/1 -> Matrix Multiply2/2
  Matrix Multiply2/1 -> Horizontal Matrix Concatenate 1/1
  Constant1/1 -> Skew-Symmetry Matrix (r_g)/9, Skew-Symmetry Matrix (r_g)/5, Skew-Symmetry Matrix (r_g)/1
  Gain/1 -> Skew-Symmetry Matrix (r_g)/2
  Gain1/1 -> Skew-Symmetry Matrix (r_g)/7
  Gain2/1 -> Skew-Symmetry Matrix (r_g)/6
  CGz/1 -> Skew-Symmetry Matrix (r_g)/4, Gain/1
  CGx/1 -> Skew-Symmetry Matrix (r_g)/8, Gain2/1
  CGy/1 -> Gain1/1, Skew-Symmetry Matrix (r_g)/3
  Matrix Multiply/1 -> Horizontal Matrix Concatenate 2/1, Gain3/1
  Gain3/1 -> Horizontal Matrix Concatenate 1/2
  Skew-Symmetry Matrix (r_g)/1 -> Matrix Multiply/2
  Constant2/1 -> Horizontal Matrix Concatenate 2/2
  Horizontal Matrix Concatenate 1/1 -> Vertical Matrix Concatenate/1
  Horizontal Matrix Concatenate 2/1 -> Vertical Matrix Concatenate/2
  Vertical Matrix Concatenate/1 -> Add/1, Display/1
  Hull Added mass/1 -> Add/2, SOURCE: Karine Chen's Added Mass Calculations/1
  Add/1 -> Matrix Multiply3/1
  Matrix Multiply3/1 -> Scope/1, Out1/1
  Body and Angular Accl/1 -> Demux/1
  Constant3/1 -> Mux/1
  Demux/1 -> Terminator/1
  Demux/2 -> Mux/2
  Demux/3 -> Mux/3
  Demux/4 -> Mux/4
  Demux/5 -> Mux/5
  Demux/6 -> Mux/6
  Mux/1 -> Matrix Multiply3/2
  2022 Hull Added mass/1 -> SOURCE: Karine Chen's Added Mass Calculations1/1, Add/3

== system hps/Plant/Hull Forces/Hull Lift//Drag ==
  note: Source of Equations:
      | Submarine Dynamic Modeling, by
      | Dr Peter Ridley Julien Fontan and Dr Peter Corke
      |
      | Part: Hydrodynamic forces and moments
  note: I think the submarine frontal area is wrong
  "Submarine Velocity (Body Axis) " : Inport
  "AOA, Side Slip" : Inport  Port=2
  Constant : Constant  Value=0
  Force Exerted due to Drag (Body Axis) : Subsystem
  Force Exerted due to Lift (Body Axis) : Subsystem
  Mux : Mux
  Sum : Sum
  "Force due to Lift, Drag" : Outport  VectorParamsAs1DForOutWhenUnconnected=off
  wires:
  Force Exerted due to Drag (Body Axis)/1(Drag Forces in Body Axis) -> Sum/1
  Force Exerted due to Lift (Body Axis)/1(Lift Forces in Body Axis) -> Sum/2
  "AOA, Side Slip"/1 -> Force Exerted due to Drag (Body Axis)/2(AOA and Side Slip), Force Exerted due to Lift (Body Axis)/2(AOA and Side Slip)
  "Submarine Velocity (Body Axis) "/1 -> Force Exerted due to Lift (Body Axis)/1(Marine Velocities in Body Axis), Force Exerted due to Drag (Body Axis)/1(Marine Velocities in Body Axis)
  Sum/1 -> Mux/1
  Mux/1 -> "Force due to Lift, Drag"/1
  Constant/1 -> Mux/4, Mux/3, Mux/2

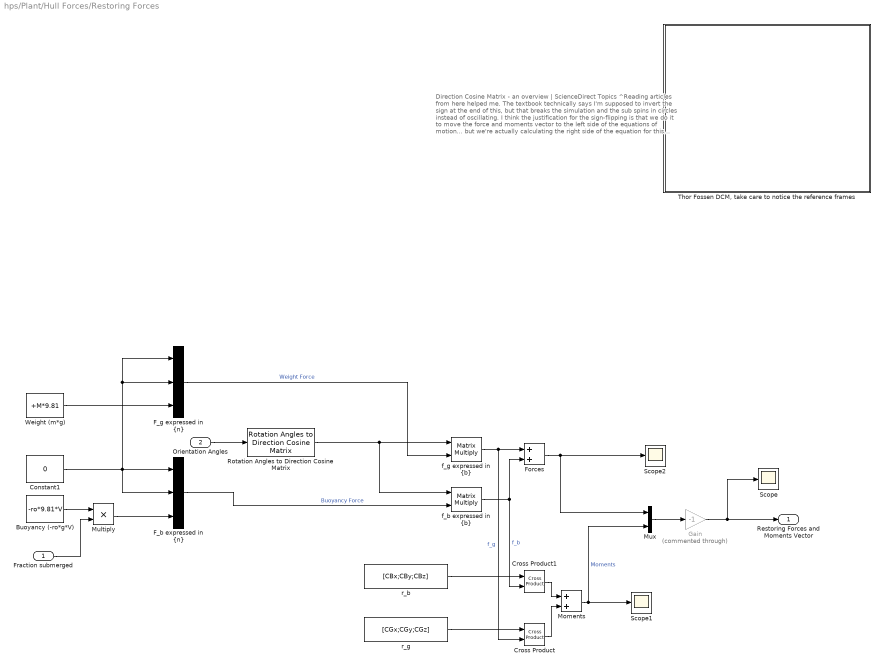
== system hps/Plant/Hull Forces/Restoring Forces ==
  note: Direction Cosine Matrix - an overview | ScienceDirect Topics
      |
      | ^Reading articles from here helped me.
      |
      | The textbook technically says I'm supposed to invert the sign at the end of this, but that breaks the simulation and the sub spins in circles instead of oscillating. I think the justification for the sign-flipping is that we do it to move the force and moments vector to the left side of the equations of motion... but we're actually calculating the right side of the equation for this model so I shouldn't flip the sign.
  "Fraction submerged " : Inport
  Orientation Angles : Inport  Port=2
  Buoyancy (-ro*g*V) : Constant  Value=-ro*9.81*V
  Constant1 : Constant  Value=0
  Cross Product : vrlib/Utilities/Cross Product
  Cross Product1 : vrlib/Utilities/Cross Product
  "F_b expressed in {n}" : Mux  Inputs=3
  "F_g expressed in {n}" : Mux  Inputs=3
  Forces : Sum
  Gain : Gain  Commented=through  Gain=-1
  Moments : Sum
  Multiply : Product
  Mux : Mux  Inputs=2
  Rotation Angles to Direction Cosine Matrix : sharedtransform/Rotation Angles to Direction Cosine Matrix  rotationOrder=XYZ  aMode=aMode
      settings: SourceProductBaseCode=AE,PW,DR,MT,UV,VE
  Scope : Scope
  Scope1 : Scope
  Scope2 : Scope
  "Thor Fossen DCM, take care to notice the reference frames" : Subsystem
      mask Display: image('$imagefile'); % Use "Edit Image" on toolstrip to change.
  Weight (m*g) : Constant  Value=+M*9.81
  "f_b expressed in {b}" : Product  Multiplication=Matrix(*)
  "f_g expressed in {b}" : Product  Multiplication=Matrix(*)
  r_b : Constant  Value=[CBx;CBy;CBz]
  r_g : Constant  Value=[CGx;CGy;CGz]
  Restoring Forces and Moments Vector : Outport
  wires:
  "Fraction submerged "/1 -> Multiply/2
  Multiply/1 -> "F_b expressed in {n}"/3
  Buoyancy (-ro*g*V)/1 -> Multiply/1
  Constant1/1 -> "F_b expressed in {n}"/2, "F_g expressed in {n}"/1, "F_g expressed in {n}"/2, "F_b expressed in {n}"/1
  Weight (m*g)/1 -> "F_g expressed in {n}"/3
  Gain/1 -> Restoring Forces and Moments Vector/1, Scope/1
  Rotation Angles to Direction Cosine Matrix/1 -> "f_b expressed in {b}"/1, "f_g expressed in {b}"/1
  Orientation Angles/1 -> Rotation Angles to Direction Cosine Matrix/1
  Moments/1 -> Scope1/1, Mux/2  "Moments"
  Cross Product1/1 -> Moments/1
  Cross Product/1 -> Moments/2
  "f_g expressed in {b}"/1 -> Forces/1, Cross Product/2  "f_g"
  "f_b expressed in {b}"/1 -> Cross Product1/2, Forces/2  "f_b"
  r_b/1 -> Cross Product1/1
  Mux/1 -> Gain/1
  "F_b expressed in {n}"/1 -> "f_b expressed in {b}"/2  "Buoyancy Force"
  Forces/1 -> Scope2/1, Mux/1
  "F_g expressed in {n}"/1 -> "f_g expressed in {b}"/2  "Weight Force"
  r_g/1 -> Cross Product/1

== system hps/Plant/6dof/Euler to VR/Axis Angle Vector ==
  e0 : Inport
  2 : Gain  Gain=2  SaturateOnIntegerOverflow=on  OutDataTypeStr=Inherit: Same as input  ParamDataTypeStr=Inherit: Same as input
  Concatenate : Concatenate
  Demux : Demux  Outputs=[1 3 ]
      settings: DisplayOption=none
  Product : Product  Inputs=*/  InputSameDT=on  SaturateOnIntegerOverflow=on  OutDataTypeStr=Inherit: Same as first input
  Trigonometric Function : Trigonometry
  Trigonometric Function2 : Trigonometry  Operator=acos
  e0_norm : Outport  VectorParamsAs1DForOutWhenUnconnected=off
  wires:
  Demux/1 -> Trigonometric Function2/1
  Demux/2 -> Product/1
  Concatenate/1 -> e0_norm/1
  Product/1 -> Concatenate/1
  2/1 -> Concatenate/2
  Trigonometric Function/1 -> Product/2
  Trigonometric Function2/1 -> Trigonometric Function/1, 2/1
  e0/1 -> Demux/1

== system hps/Plant/6dof/Euler to VR/Quaternion Normalization ==
  e0 : Inport
  1/2 : Gain  Gain=1/2  SaturateOnIntegerOverflow=on  OutDataTypeStr=Inherit: Same as input  ParamDataTypeStr=Inherit: Same as input
  Concatenate : Concatenate
  Demux : Demux  Outputs=[1 3]
      settings: DisplayOption=none
  Product : Product  InputSameDT=on  SaturateOnIntegerOverflow=on  OutDataTypeStr=Inherit: Same as first input
  Trigonometric Function : Trigonometry
  Trigonometric Function1 : Trigonometry  Operator=cos
  e0_norm : Outport  VectorParamsAs1DForOutWhenUnconnected=off
  wires:
  Trigonometric Function1/1 -> Concatenate/1
  Demux/2 -> Product/2
  Demux/1 -> 1/2/1
  Concatenate/1 -> e0_norm/1
  Product/1 -> Concatenate/2
  Trigonometric Function/1 -> Product/1
  1/2/1 -> Trigonometric Function1/1, Trigonometric Function/1
  e0/1 -> Demux/1

== system hps/Plant/6dof/Euler to VR/Quaternion Normalization1 ==
  e0 : Inport
  1/2 : Gain  Gain=1/2  SaturateOnIntegerOverflow=on  OutDataTypeStr=Inherit: Same as input  ParamDataTypeStr=Inherit: Same as input
  Concatenate : Concatenate
  Demux : Demux  Outputs=[1 3]
      settings: DisplayOption=none
  Product : Product  InputSameDT=on  SaturateOnIntegerOverflow=on  OutDataTypeStr=Inherit: Same as first input
  Trigonometric Function : Trigonometry
  Trigonometric Function1 : Trigonometry  Operator=cos
  e0_norm : Outport  VectorParamsAs1DForOutWhenUnconnected=off
  wires:
  e0/1 -> Demux/1
  1/2/1 -> Trigonometric Function/1, Trigonometric Function1/1
  Trigonometric Function/1 -> Product/1
  Product/1 -> Concatenate/2
  Concatenate/1 -> e0_norm/1
  Demux/1 -> 1/2/1
  Demux/2 -> Product/2
  Trigonometric Function1/1 -> Concatenate/1

== system hps/Plant/6dof/Euler to VR/Quaternion Normalization2 ==
  e0 : Inport
  1/2 : Gain  Gain=1/2  SaturateOnIntegerOverflow=on  OutDataTypeStr=Inherit: Same as input  ParamDataTypeStr=Inherit: Same as input
  Concatenate : Concatenate
  Demux : Demux  Outputs=[1 3]
      settings: DisplayOption=none
  Product : Product  InputSameDT=on  SaturateOnIntegerOverflow=on  OutDataTypeStr=Inherit: Same as first input
  Trigonometric Function : Trigonometry
  Trigonometric Function1 : Trigonometry  Operator=cos
  e0_norm : Outport  VectorParamsAs1DForOutWhenUnconnected=off
  wires:
  Trigonometric Function1/1 -> Concatenate/1
  Demux/2 -> Product/2
  Demux/1 -> 1/2/1
  Concatenate/1 -> e0_norm/1
  Product/1 -> Concatenate/2
  Trigonometric Function/1 -> Product/1
  1/2/1 -> Trigonometric Function1/1, Trigonometric Function/1
  e0/1 -> Demux/1

== system hps/Plant/Hull Forces/Hull Inertia/M = Rigid Body Inertia + Added Mass Inertia ==

== system hps/Plant/Hull Forces/Hull Inertia/Subsystem ==

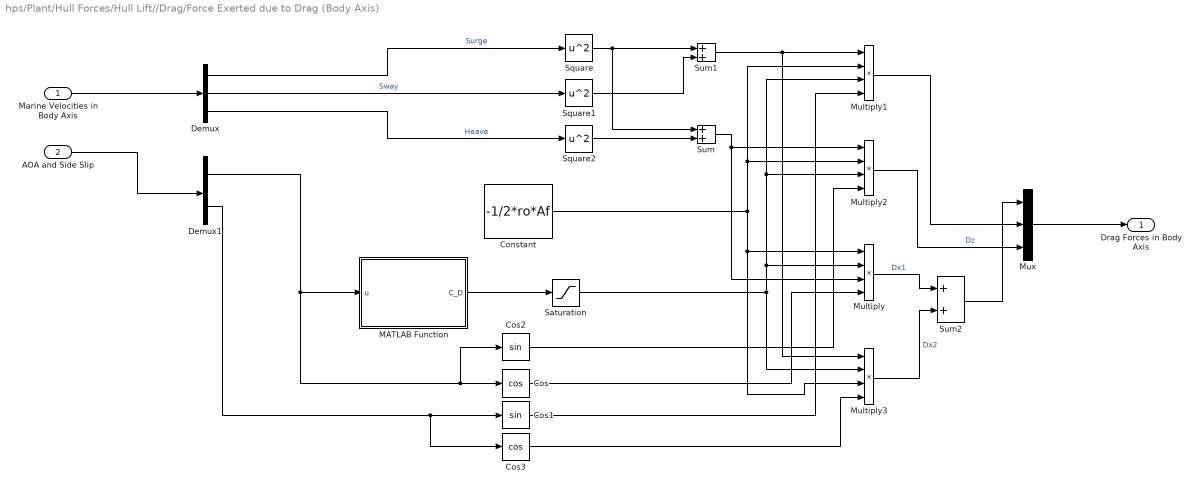
== system hps/Plant/Hull Forces/Hull Lift//Drag/Force Exerted due to Drag (Body Axis) ==
  Marine Velocities in Body Axis : Inport
  AOA and Side Slip : Inport  Port=2
  Constant : Constant  Value=-1/2*ro*Af  mask{ro=997, Af=0.22}
      mask prompts: ro "Density of Water"; Af "Submarine Frontal Area"
      mask DialogControl DescGroupVar Prompt: Input
      mask DialogControl DescTextVar Prompt: Enter the following values :
  Cos : Trigonometry  Operator=cos
  Cos1 : Trigonometry
  Cos2 : Trigonometry
  Cos3 : Trigonometry  Operator=cos
  Demux : Demux  Outputs=3
  Demux1 : Demux  Outputs=2
  MATLAB Function : MATLAB Function  TreatAsAtomicUnit=on
  Multiply{,1..3} (4 alike) : Product  Inputs=4
  Mux : Mux  Inputs=3
  Saturation : Saturate  UpperLimit=73.2049  LowerLimit=-73.2049
  Square : Math  Operator=square  SignedPower=on  SaturateOnIntegerOverflow=on
  Square1 : Math  Operator=square  SignedPower=on  SaturateOnIntegerOverflow=on
  Square2 : Math  Operator=square  SignedPower=on  SaturateOnIntegerOverflow=on
  Sum : Sum
  Sum1 : Sum
  Sum2 : Sum
  Drag Forces in Body Axis : Outport  VectorParamsAs1DForOutWhenUnconnected=off
  wires:
  Saturation/1 -> Multiply/2, Multiply2/3, Multiply1/3, Multiply3/2
  Square1/1 -> Sum1/2
  Multiply1/1 -> Mux/2
  Sum2/1 -> Mux/1
  Cos3/1 -> Multiply3/4
  AOA and Side Slip/1 -> Demux1/1
  Marine Velocities in Body Axis/1 -> Demux/1
  Cos2/1 -> Multiply2/4
  Mux/1 -> Drag Forces in Body Axis/1
  Square2/1 -> Sum/2
  Demux1/2 -> Cos1/1, Cos3/1
  Demux1/1 -> MATLAB Function/1(u), Cos2/1, Cos/1
  MATLAB Function/1(C_D) -> Saturation/1
  Multiply2/1 -> Mux/3  "Dz"
  Cos/1 -> Multiply/4
  Demux/3 -> Square2/1  "Heave"
  Constant/1 -> Multiply2/2, Multiply1/2, Multiply/1, Multiply3/3
  Multiply3/1 -> Sum2/2  "Dx2"
  Sum/1 -> Multiply/3, Multiply2/1
  Demux/1 -> Square/1  "Surge"
  Multiply/1 -> Sum2/1  "Dx1"
  Sum1/1 -> Multiply1/1, Multiply3/1
  Cos1/1 -> Multiply1/4
  Demux/2 -> Square1/1  "Sway"
  Square/1 -> Sum1/1, Sum/1

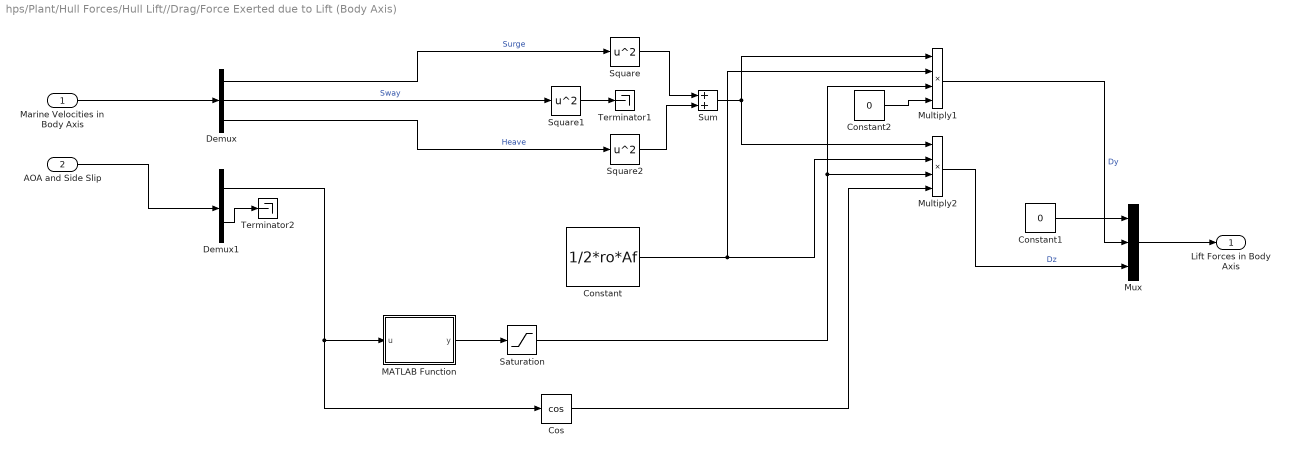
== system hps/Plant/Hull Forces/Hull Lift//Drag/Force Exerted due to Lift (Body Axis) ==
  Marine Velocities in Body Axis : Inport
  AOA and Side Slip : Inport  Port=2
  Constant : Constant  Value=1/2*ro*Af  mask{ro=997, Af=0.22}
      mask prompts: ro "Density of Water"; Af "Submarine Frontal Area"
      mask DialogControl DescGroupVar Prompt: Input
      mask DialogControl DescTextVar Prompt: Enter the following values :
  Constant1 : Constant  Value=0
  Constant2 : Constant  Value=0
  Cos : Trigonometry  Operator=cos
  Demux : Demux  Outputs=3
  Demux1 : Demux  Outputs=2
  MATLAB Function : MATLAB Function  TreatAsAtomicUnit=on
  Multiply1 : Product  Inputs=4
  Multiply2 : Product  Inputs=4
  Mux : Mux  Inputs=3
  Saturation : Saturate  UpperLimit=73.2049  LowerLimit=-73.2049
  Square : Math  Operator=square  SignedPower=on  SaturateOnIntegerOverflow=on
  Square1 : Math  Operator=square  SignedPower=on  SaturateOnIntegerOverflow=on
  Square2 : Math  Operator=square  SignedPower=on  SaturateOnIntegerOverflow=on
  Sum : Sum
  Terminator1 : Terminator
  Terminator2 : Terminator
  Lift Forces in Body Axis : Outport  VectorParamsAs1DForOutWhenUnconnected=off
  wires:
  Saturation/1 -> Multiply2/3, Multiply1/3
  Constant2/1 -> Multiply1/4
  Multiply2/1 -> Mux/3  "Dz"
  Constant1/1 -> Mux/1
  Cos/1 -> Multiply2/4
  Square/1 -> Sum/1
  Demux/2 -> Square1/1  "Sway"
  Demux/1 -> Square/1  "Surge"
  Sum/1 -> Multiply1/1, Multiply2/1
  Constant/1 -> Multiply1/2, Multiply2/2
  Multiply1/1 -> Mux/2  "Dy"
  Demux/3 -> Square2/1  "Heave"
  MATLAB Function/1(y) -> Saturation/1
  Demux1/1 -> MATLAB Function/1(u), Cos/1
  Square2/1 -> Sum/2
  Mux/1 -> Lift Forces in Body Axis/1
  Marine Velocities in Body Axis/1 -> Demux/1
  AOA and Side Slip/1 -> Demux1/1
  Square1/1 -> Terminator1/1
  Demux1/2 -> Terminator2/1

== system hps/Plant/Hull Forces/Restoring Forces/Thor Fossen DCM, take care to notice the reference frames ==

== matlab function hps/Plant/Hull Forces/Hull Lift//Drag/Force Exerted due to Lift (Body Axis)/MATLAB Function ==
  data: u input; y output
function y = fcn(u)
if u>pi/2
    u = u-pi;
elseif u < -pi/2
    u = u + pi;
end

y = .0662 * (u) + 0;

== matlab function hps/Plant/Fin (control) Forces/2021 Single Fin Drag/Area ==
  data: finbeam input; A output; semi_major input; semi_minor input
function A = fcn(finbeam, semi_major, semi_minor)
fun = @(r) r^3 * 2*sqrt(semi_minor^2 * (1 - (r-(finbeam/2 - semi_major)^2)/semi_major^2));
A = integral(fun, 0.5*finbeam - semi_major, 0.5*finbeam);

== matlab function hps/Plant/Fin (control) Forces/Single Fin Lift/MATLAB Function ==
  data: u input; y output
function y = fcn(u)
if u>pi/2
    u = u-pi;
elseif u < -pi/2
    u = u + pi;
end

y = .108 * (u) + 0;

== matlab function hps/Plant/Fin (control) Forces/Single Fin Drag/MATLAB Function1 ==
  data: u input; C_D output
function C_D = Calculate_Drag_Coeff(u)
if u>pi/2
    u = u-pi;
elseif u < -pi/2
    u = u + pi;
end
C_D = 0.000155*(u.^2) - 0.0000000388 * (u) + 0.00655;

== matlab function hps/Plant/Hull Forces/Hull Lift//Drag/Force Exerted due to Drag (Body Axis)/MATLAB Function ==
  data: u input; C_D output
function C_D = Calculate_Drag_Coeff(u)
if u>pi/2
    u = u-pi;
elseif u < -pi/2
    u = u + pi;
end
C_D = 0.0003*(u.^2) + 0.00004 * (u) + 0.0011;
